simulink model "examples5and6"  (R2023b)
settings: Solver=VariableStepAuto  StartTime=0.0  StopTime=10.0  RelTol=1e-3
model workspace (MAT data in the model file):
  c = 5
  m = 25
undefined symbols (not defined in the file): x
settings Model: Creator=ray  LastModifiedBy=ray

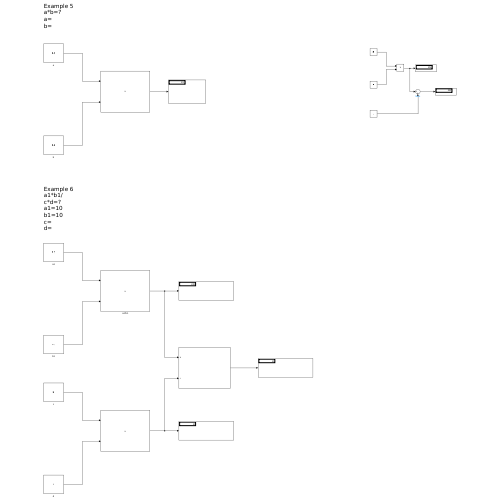
[thumbnail: Simulink's stored preview of the top-level diagram]
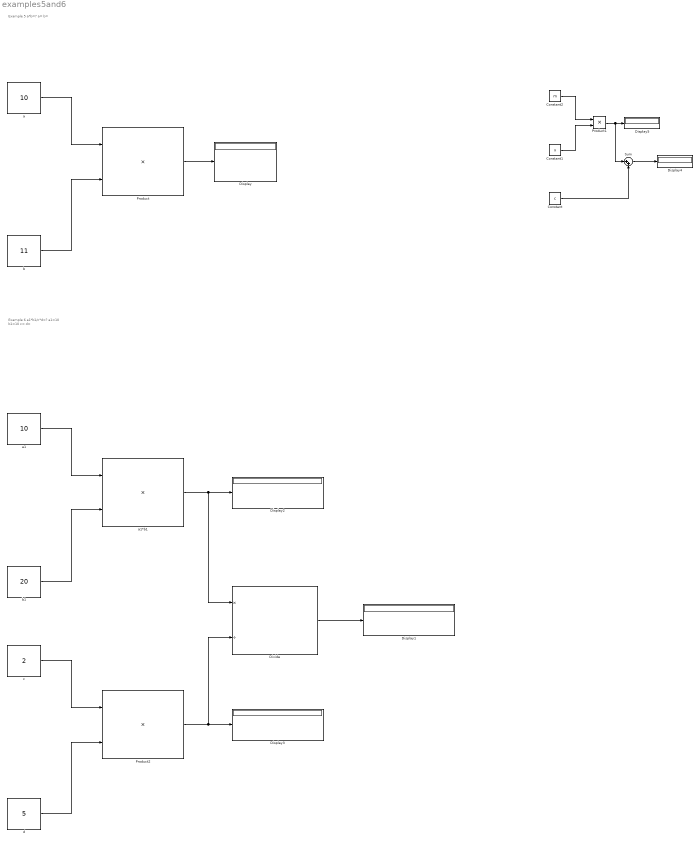
== system examples5and6 ==
  note: Example 5
      | a*b=?
      | a=
      | b=
  note: Example 6
      | a1*b1/c*d=?
      | a1=10
      | b1=10
      | c=
      | d=
  Constant : Constant  Value=c
  Constant1 : Constant  Value=x
  Constant2 : Constant  Value=m
  Display{,1..5} (6 alike) : Display
  Divide : Product  Inputs=*/
  Product : Product
  Product1 : Product
  Product2 : Product
  Sum : Sum  Inputs=|++
  a : Constant  Value=10
  a1 : Constant  Value=10
  a1*b1 : Product
  b : Constant  Value=11
  b1 : Constant  Value=20
  c : Constant  Value=2
  d : Constant  Value=5
  wires:
  a/1 -> Product/1
  b/1 -> Product/2
  Product/1 -> Display/1
  a1/1 -> a1*b1/1
  b1/1 -> a1*b1/2
  d/1 -> Product2/2
  c/1 -> Product2/1
  a1*b1/1 -> Divide/1, Display2/1
  Product2/1 -> Display3/1, Divide/2
  Divide/1 -> Display1/1
  Constant2/1 -> Product1/1
  Constant1/1 -> Product1/2
  Product1/1 -> Display5/1, Sum/1
  Constant/1 -> Sum/2
  Sum/1 -> Display4/1
